simulink model "tpfinal"  (R2020a)
settings: Solver=VariableStepAuto  StartTime=0.0  StopTime=5000.0  RelTol=1e-3
settings Model: Creator=emili  LastModifiedBy=emili

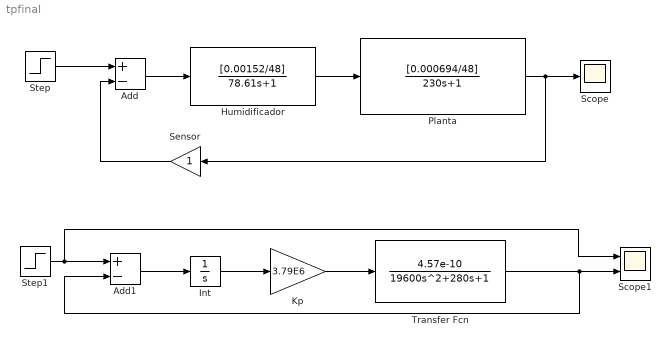
== system tpfinal ==
  Add : Sum  Inputs=+-
  Add1 : Sum  Inputs=+-
  Humidificador : TransferFcn  Numerator=[0.00152/48]  Denominator=[78.61 1]
  Int : Integrator
  Kp : Gain  Gain=3.79E6
  Planta : TransferFcn  Numerator=[0.000694/48]  Denominator=[230 1]
  Scope : Scope
  Scope1 : Scope  NumInputPorts=2
  Sensor : Gain
  Step : Step  Time=0.001  After=10  SampleTime=0
  Step1 : Step  Time=0.001  SampleTime=0
  Transfer Fcn : TransferFcn  Numerator=[ 4.57e-10]  Denominator=[19600 280 1]
  wires:
  Step/1 -> Add/1
  Humidificador/1 -> Planta/1
  Planta/1 -> Scope/1, Sensor/1
  Sensor/1 -> Add/2
  Add/1 -> Humidificador/1
  Step1/1 -> Scope1/1, Add1/1
  Kp/1 -> Transfer Fcn/1
  Transfer Fcn/1 -> Scope1/2, Add1/2
  Add1/1 -> Int/1
  Int/1 -> Kp/1
